simulink model "motorsimulink"  (R2022a)
settings: Solver=VariableStepAuto  StartTime=0.0  StopTime=0.01  RelTol=1e-3
values from neighbouring files (symbols this model uses):
  L = 0.0238    [parametrosmotor.m]
  R = 2.06    [parametrosmotor.m]
undefined symbols (not defined in the file or in its folder): C
settings Model: Creator=fermo  LastModifiedBy=fermo

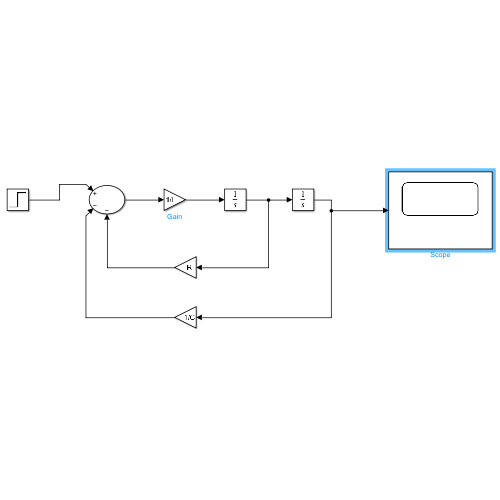
[thumbnail: Simulink's stored preview of the top-level diagram]
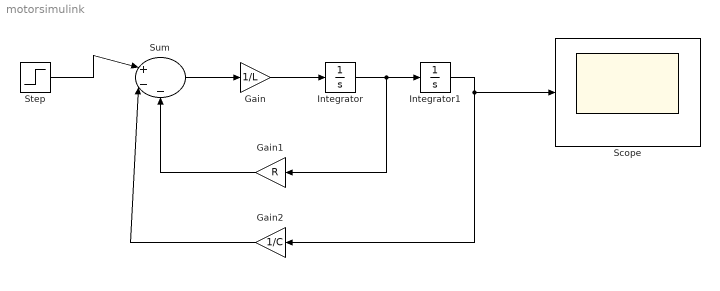
== system motorsimulink ==
  Gain : Gain  Gain=1/L
  Gain1 : Gain  Gain=R
  Gain2 : Gain  Gain=1/C
  Integrator : Integrator
  Integrator1 : Integrator
  Scope : Scope
  Step : Step  Time=0  After=5  SampleTime=0
  Sum : Sum  Inputs=|+--
  wires:
  Gain/1 -> Integrator/1
  Integrator/1 -> Gain1/1, Integrator1/1
  Integrator1/1 -> Gain2/1, Scope/1
  Gain1/1 -> Sum/3
  Gain2/1 -> Sum/2
  Sum/1 -> Gain/1
  Step/1 -> Sum/1
